simulink model "Exp2_SolucionDiferencial"  (R2023a)
settings: Solver=ode8  StartTime=0.0  StopTime=10.0  FixedStep=0.01  RelTol=1e-3
values from neighbouring files (symbols this model uses):
  b = 0.2    [Experimento2.m]
  k = 1.5    [Experimento2.m]
  m = 2    [Experimento2.m]
settings Model: Creator=carlo  LastModifiedBy=carlo

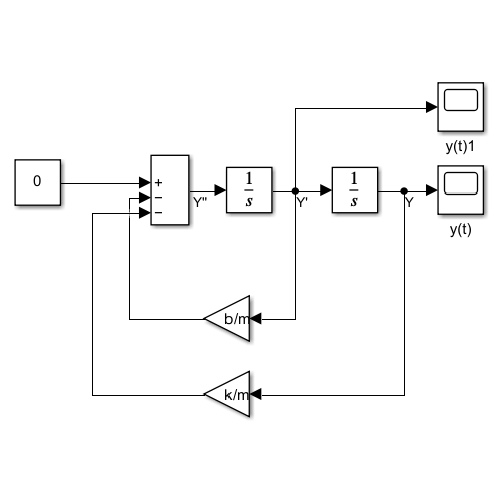
[thumbnail: Simulink's stored preview of the top-level diagram]
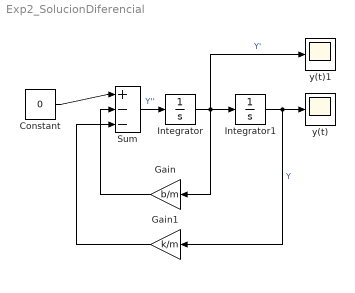
== system Exp2_SolucionDiferencial ==
  Constant : Constant  Value=0
  Gain : Gain  Gain=b/m
  Gain1 : Gain  Gain=k/m
  Integrator : Integrator
  Integrator1 : Integrator  InitialCondition=2
  Sum : Sum  Inputs=|+--
  y(t) : Scope
  y(t)1 : Scope
  wires:
  Integrator/1 -> y(t)1/1, Gain/1, Integrator1/1  "Y'"
  Integrator1/1 -> Gain1/1, y(t)/1  "Y"
  Sum/1 -> Integrator/1  "Y''"
  Gain/1 -> Sum/2
  Gain1/1 -> Sum/3
  Constant/1 -> Sum/1
